simulink model "pwm_block"  (R2017a)
settings: Solver=VariableStepAuto  StartTime=0.0  StopTime=10.0  RelTol=1e-3
values from neighbouring files (symbols this model uses):
  Tpwm_val = 1e-3    (= 0.001)    [ss_value.m]
  Ts_val = 1.1e-2    (= 0.011)    [ss_value.m]
undefined symbols (not defined in the file or in its folder): alpha_ss
settings Model: Creator=brunolnetto  LastModifiedBy=brunolnetto

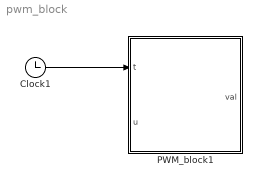
== system pwm_block ==
  Clock1 : Clock
  PWM_block1 : MATLAB Function  TreatAsAtomicUnit=on
  wires:
  Clock1/1 -> PWM_block1/1(t)

== matlab function pwm_block/PWM_block1 ==
  data: t input; u input; val output; alpha_ss parameter; Tpwm_val parameter; Ts_val parameter
function val = pwm_signal(t, u, alpha_ss, Tpwm_val, Ts_val)
    % Evaluation of external functions
    coder.extrinsic('evalin');
    coder.extrinsic('place');
    coder.extrinsic('assigin');

    % Static variable
    persistent t0;
    
    if(isempty(t0))
        t0 = 0;
    end
    
    % Minimum and maximum values
    min_val = u(1);
    max_val = u(2);
    
    % PWM generation
    if(t == 0)
        t0 = 0;
    end
    
    if(t - t0 > Tpwm_val)
        t0 = t;
    end
    
    % Inner time interval
    t_i = t - t0;
    
    if(t_i <= alpha_ss*Tpwm_val)
        val = max_val;
    else
        val = min_val;
    end
    
    n = floor(Ts_val/Tpwm_val);
    if(Ts_val - Tpwm_val*n > 0)
        phi_aug = evalin('base', 'phi_aug');
        gamma_aug = evalin('base', 'gamma_aug');
        poles_d = evalin('base', 'poles_d');
        
        K_aug = place(phi_aug, gamma_aug, poles_d);

        assigin('base', 'K_aug', K_aug);
    end
end
